simulink model "exampleRadiationInclinedSurface"  (Simulink 7.6)
settings: Solver=VariableStepDiscrete  StartTime=0.0  StopTime=24*3600  RelTol=1e-3
libraries: carnot x3
settings Model: Creator=drhf  LastModifiedBy=drhf

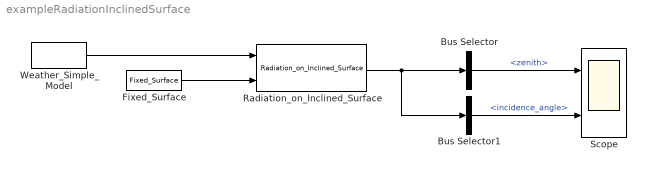
== system exampleRadiationInclinedSurface ==
  Bus Selector : BusSelector  OutputSignals=Zenith_Angle,Azimuth_Angle  OutputAsBus=on
  Bus Selector1 : BusSelector  OutputSignals=Incidence_Angle_sun,Incidence_Angle_longitudinal,Incidence_Angle_transversal  OutputAsBus=on
  Fixed_Surface : carnot/Weather/Fixed_Surface  SystemSampleTime=-1  colangle=30  colazi=0  colrot=0
  Radiation_on_Inclined_Surface : carnot/Weather/Radiation_on_Inclined_Surface  SystemSampleTime=-1  sky=Perez 1990  reflect=0.2
  Scope : Scope  NumInputPorts=2
      settings: YMin=-5~-5  YMax=5~5
  Weather_Simple_Model : carnot/Weather/Weather_Simple_Model  SystemSampleTime=-1  lat=60  Ibn=900  Idg=100  tamb=5  deltaTsky=-6  rh=50  precip="10e-3/24/3600           % 10 mm in 24 h"  cloud=0.125  p=1013e2  vw=1  wdir=270
  wires:
  Weather_Simple_Model/1 -> Radiation_on_Inclined_Surface/1
  Fixed_Surface/1 -> Radiation_on_Inclined_Surface/2
  Radiation_on_Inclined_Surface/1 -> Bus Selector1/1, Bus Selector/1
  Bus Selector/1 -> Scope/1  "<zenith>"
  Bus Selector1/1 -> Scope/2  "<incidence_angle>"
